simulink model "ACDCMG_woPV"  (R2020b)
settings: Solver=FixedStepAuto  StartTime=0.0  StopTime=0.2  FixedStep=Ts  MaxStep=1e-2  RelTol=1e-3
InitFcn:
  | Set_parameters_R2018
undefined symbols (not defined in the file): D1, D_invs, Delta, dis11, dis14, dis2, dis3, dis4, dis5, dis6, dis8, DiscIntNeverNeededParam, ee_sli_rtmsupport, fn, Fnom, gcbh, H_invs, Ion, Lithium, max_min, P_Load_3, P_nom_inv, Pnom_T1, Pnom_T2, Pnom_T3, Ql_Load_3, R_Load_9, R_Load_DC, Rl, Rls, S, sigbuilder_block, Ts, Ts_Control, Ts_Power, V1_LL_T3, VnInv, Vnom_DC, Vnom_Diesel, Vnom_prim, Vnom_sec, Vnom_ter_AC_DC, Xl, Xls
libraries: powerlib x238, powerlib_meascontrol x103, powerlib_extras x55, simulink x21, pid_lib x4, eeGeneralControl x2, re_lib x1, electricdrivelib x1, eeSinusoidalMeasurementV2 x1, eePowerMeasurement x1
(part 1 of 9)
settings Model: Creator=Leony  LastModifiedBy=Fangyuan
settings SolverCC: ZeroCrossAlgorithm=Adaptive  SolverResetMethod=Robust
settings DataIOCC: LimitDataPoints=on  SaveFormat=Array  ReturnWorkspaceOutputs=off
settings OptimizationCC: LifeSpan=inf
settings DebuggingCC: AlgebraicLoopMsg=none  UnderspecifiedInitializationDetection=Classic  MergeDetectMultiDrivingBlocksExec=none  IgnoredZcDiagnostic=none  SolverPrmCheckMsg=warning  AllowSymbolicDim=off  SFUnexpectedBacktrackingDiag=warning  SFNoUnconditionalDefaultTransitionDiag=warning  SFExecutionAtInitializationDiag=none  ArithmeticOperatorsInVariantConditions=warning
settings HardwareCC: ProdBitPerPointer=32  ProdBitPerSizeT=32  ProdBitPerPtrDiffT=32  ProdLargestAtomicFloat=None  ProdIntDivRoundTo=Undefined  ProdEndianess=Unspecified  ProdWordSize=32  ProdHWDeviceType=32-bit Generic
settings ModelReferenceCC: PropagateSignalLabelsOutOfModel=off
settings SFSimCC: SimUseLocalCustomCode=off  CustomCodeUndefinedFunction=UseInterfaceOnly
settings RTWCC: RTWUseLocalCustomCode=off
settings CodeAppCC: StateflowObjectComments=on
settings GRTTargetCC: TargetLangStandard=C89/C90 (ANSI)
settings ConfigComp: CovMetricSettings=dw  CovSaveCumulativeToWorkspaceVar=on  CovSaveSingleToWorkspaceVar=on  CovExternalEMLEnable=off
settings SimscapeCC: SimscapeNormalizeSystem=off

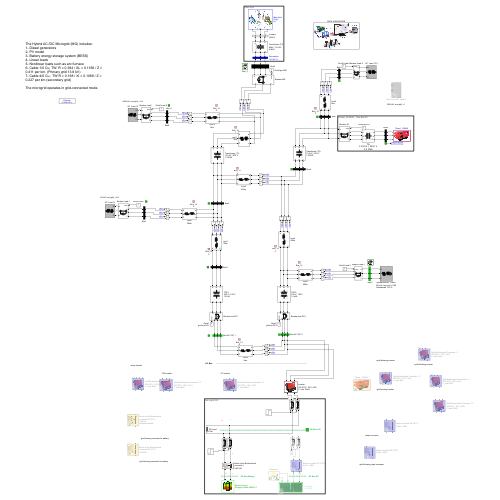
[thumbnail: Simulink's stored preview of the top-level diagram]
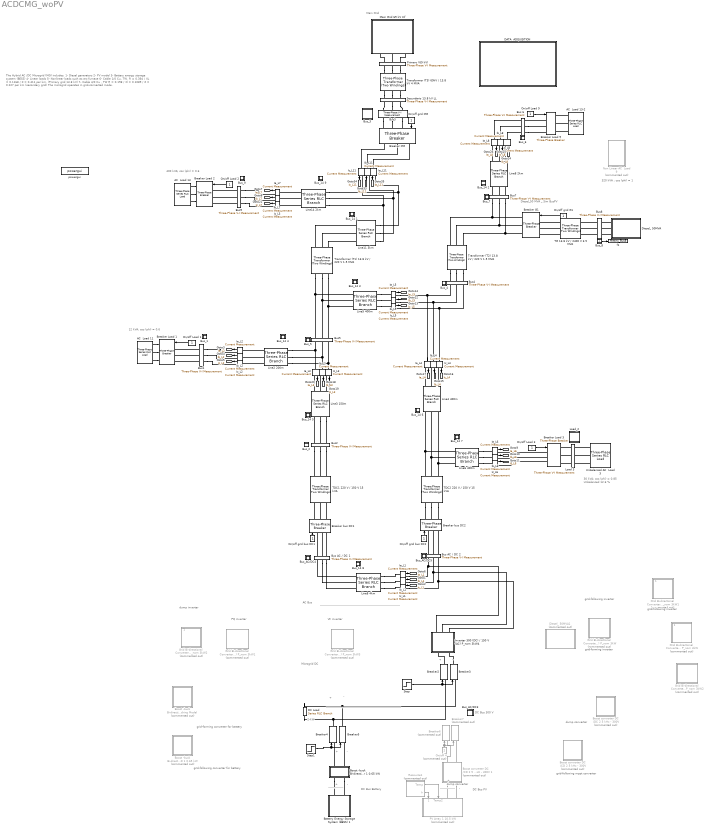
== system ACDCMG_woPV ==
  note: dump inverter
  note: PQ inverter
  note: VF inverter
  note: grid-following inverter
  note: grid-following converter for battery
  note: grid-forming inverter
  note: dump converter
  note: grid-following mppt converter
  note: Main Grid
  note: The Hybrid AC /DC Microgrid (MG) includes:
      | 1- Diesel generators
      | 2- PV model
      | 3- Battery energy storage system (BESS)
      | 4- Linear loads
      | 5- Nonlinear loads such as arc furnace
      | 6- Cable 1/0 Cu, TW. R = 0.394 / XL = 0.1168 / Z = 0.411 per km. (Primary grid 13.8 kV)
      | 7- Cable 4/0 Cu , TW R = 0.198 / Xl = 0.1089 / Z = 0.227 per km (secondary grid)
      |
      | The microgrid operates in grid-connected mode.
  note: --------------------------------------------------------------------------------
  note: AC Bus
  note: Diesel_50 MVA _ Sim BusPV
  note: 30 kVA; cos (phi) = 0.85
      | Unbalanced 12.6 %
  note: 320 kVA ; cos (phi) = 1
  note: 12 kVA; cos (phi) = 0.6
  note: 400 kVA; cos (phi) = 0.6
  note: grid-forming converter for battery
  note: -
  note: ---------------------------------------------------------------------------
  note: -
  note: DC Bus Battery
  note: DC Bus 300 V
  note: +
  note: ---------------
  note: -
  note: -
  note: +
  note: +
  note: 2 kW
  note: +
  note: ---------------
  note: dump converter
  note: DC Bus PV
  note: +
  note: -
  note: Microgrid DC
  note: grid-following inverter
    Ic_L{3..4,8,11} (4 alike) : powerlib/Measurements/Current Measurement  PhasorSimulation=off  OutputType=Complex  PSBequivalent=0
  "  PV Array 1 10.5 kW" : Subsystem  Commented=on
      mask Display: image(imread('Icons\PV.png'));
  " Bus3" : powerlib/Measurements/Three-Phase V-I Measurement  VoltageMeasurement=phase-to-ground  SetLabelV=on  LabelV=Vabc_LL_Bus3  Vpu=off  VpuLL=off  CurrentMeasurement=yes  SetLabelI=on  LabelI=Iabc_LL_Bus3  Ipu=off  Pbase=100e6  Vbase=500e3  OutputType=Complex  PhasorSimulation=off  PSBequivalent=0
  AC  Load 11 : powerlib/Elements/Three-Phase Series RLC Load  LConnTagsString=A|B|C  Configuration=Y (grounded)  NominalVoltage=Vnom_sec  Vabc=[1e3 1e3 1e3]  Vabcp=[1e3 1e3 1e3]  NominalFrequency=Fnom  UnbalancedPower=off  ActivePower=P_Load_11  InductivePower=Ql_Load_11  CapacitivePower=0  Pabc=[10e3 9e3 11e3]  QLabc=[100 90 110]  QCabc=[100 90 110]  Pabcp=[10e3 9e3 11e3]  QLabcp=[100 90 110]  QCabcp=[100 90 110]  Measurements=None  LoadType=constant Z
  AC  Load 13 : powerlib/Elements/Three-Phase Series RLC Load  LConnTagsString=A|B|C  Configuration=Y (grounded)  NominalVoltage=Vnom_prim  Vabc=[1e3 1e3 1e3]  Vabcp=[1e3 1e3 1e3]  NominalFrequency=Fnom  UnbalancedPower=off  ActivePower=P_Load_13  InductivePower=Ql_Load_13  CapacitivePower=0  Pabc=[10e3 9e3 11e3]  QLabc=[100 90 110]  QCabc=[100 90 110]  Pabcp=[10e3 9e3 11e3]  QLabcp=[100 90 110]  QCabcp=[100 90 110]  Measurements=None  LoadType=constant Z
  AC  Load 13-2 : powerlib/Elements/Three-Phase Series RLC Load  LConnTagsString=A|B|C  Configuration=Y (grounded)  NominalVoltage=Vnom_prim  Vabc=[1e3 1e3 1e3]  Vabcp=[1e3 1e3 1e3]  NominalFrequency=Fnom  UnbalancedPower=off  ActivePower=P_Load_15  InductivePower=Ql_Load_15  CapacitivePower=0  Pabc=[10e3 9e3 11e3]  QLabc=[100 90 110]  QCabc=[100 90 110]  Pabcp=[10e3 9e3 11e3]  QLabcp=[100 90 110]  QCabcp=[100 90 110]  Measurements=None  LoadType=constant Z
  Battery Energy Storage System (BESS) 1 : Subsystem
      mask Display: image('Icons\Battery Energy Storage System (BESS).png');
  Boost -buck Bi-directional converter 1 0.65 kW : Subsystem
      mask Display: image(imread('Icons\DC_DC_Converter.jpg'));
  Boost -buck Bi-directional converter DC /CD 1 0.65 kW : Subsystem  Commented=on
      mask Display: image(imread('Icons\DC_DC_Converter.jpg'));
  Boost -buck Bi-directional converter DC /DC 1 0.65 kW Switching Model : Subsystem  Commented=on
      mask Display: image(imread('Icons\DC_DC_Converter.jpg'));
  "Boost converter DC /CD 2 5 kHz - 300V " : Subsystem  Commented=on
      mask Display: image(imread('Icons\DC_DC_Converter.jpg'));
  Boost converter DC /CD 2 5 kHz - 300V 1 : Subsystem  Commented=on
      mask Display: image(imread('Icons\DC_DC_Converter.jpg'));
  "Boost converter DC /DC 2 5 kHz - 300V " : Subsystem  Commented=on
      mask Display: image(imread('Icons\DC_DC_Converter.jpg'));
  Breaker G1 : powerlib/Elements/Three-Phase Breaker  InitialState=closed  SwitchA=on  SwitchB=on  SwitchC=on  SwitchTimes="[4/60  10/60]"  External=on  BreakerResistance=0.001  SnubberResistance=1e6  SnubberCapacitance=inf  Measurements=None
  Breaker Load {1..3,9} (4 alike) : powerlib/Elements/Three-Phase Breaker  InitialState=closed  SwitchA=on  SwitchB=on  SwitchC=on  SwitchTimes="[4/60  10/60]"  External=on  BreakerResistance=0.001  SnubberResistance=1e6  SnubberCapacitance=inf  Measurements=None
  Breaker MG : powerlib/Elements/Three-Phase Breaker  InitialState=closed  SwitchA=on  SwitchB=on  SwitchC=on  SwitchTimes="[4/60  10/60]"  External=on  BreakerResistance=0.001  SnubberResistance=1e6  SnubberCapacitance=inf  Measurements=None
  Breaker bus DC1 : powerlib/Elements/Three-Phase Breaker  InitialState=closed  SwitchA=on  SwitchB=on  SwitchC=on  SwitchTimes="[4/60  10/60]"  External=on  BreakerResistance=0.001  SnubberResistance=1e6  SnubberCapacitance=inf  Measurements=None
  Breaker bus DC2 : powerlib/Elements/Three-Phase Breaker  InitialState=closed  SwitchA=on  SwitchB=on  SwitchC=on  SwitchTimes="[4/60  10/60]"  External=on  BreakerResistance=0.001  SnubberResistance=1e6  SnubberCapacitance=inf  Measurements=None
  Breaker{2..5} (4 alike) : powerlib/Elements/Breaker  InitialState=1  SwitchingTimes="[1/60  5/60]"  External=on  BreakerResistance=0.01  SnubberResistance=1e6  SnubberCapacitance=inf  Measurements=None  MoreParameters=on  NoBreakLoop=off
  Breaker6 : powerlib/Elements/Breaker  Commented=on  InitialState=1  SwitchingTimes="[1/60  5/60]"  External=on  BreakerResistance=0.01  SnubberResistance=1e6  SnubberCapacitance=inf  Measurements=None  MoreParameters=on  NoBreakLoop=off
  Breaker7 : powerlib/Elements/Breaker  Commented=on  InitialState=1  SwitchingTimes="[1/60  5/60]"  External=on  BreakerResistance=0.01  SnubberResistance=1e6  SnubberCapacitance=inf  Measurements=None  MoreParameters=on  NoBreakLoop=off
  Bus 6 : powerlib/Measurements/Three-Phase V-I Measurement  VoltageMeasurement=phase-to-ground  SetLabelV=on  LabelV=VabcLL_Bus_6  Vpu=off  VpuLL=off  CurrentMeasurement=yes  SetLabelI=on  LabelI=IabcLL_Bus_6  Ipu=off  Pbase=100e6  Vbase=25e3/sqrt(2)  OutputType=Complex  PhasorSimulation=off  PSBequivalent=0
  Bus AC / DC 1 : powerlib/Measurements/Three-Phase V-I Measurement  VoltageMeasurement=phase-to-ground  SetLabelV=on  LabelV=Vabc_B1_busDC1  Vpu=off  VpuLL=off  CurrentMeasurement=yes  SetLabelI=on  LabelI=Iabc_B1_busDC1  Ipu=off  Pbase=100e6  Vbase=25e3  OutputType=Complex  PhasorSimulation=off  PSBequivalent=0
  Bus AC / DC 2 : powerlib/Measurements/Three-Phase V-I Measurement  VoltageMeasurement=phase-to-ground  SetLabelV=on  LabelV=Vabc_B1_busDC2  Vpu=off  VpuLL=off  CurrentMeasurement=yes  SetLabelI=on  LabelI=Iabc_B1_busDC2  Ipu=off  Pbase=100e6  Vbase=25e3  OutputType=Complex  PhasorSimulation=off  PSBequivalent=0
  Bus1 : powerlib/Measurements/Three-Phase V-I Measurement  VoltageMeasurement=phase-to-ground  SetLabelV=on  LabelV=VabcLL_Bus_1  Vpu=off  VpuLL=off  CurrentMeasurement=yes  SetLabelI=on  LabelI=IabcLL_Bus_1  Ipu=off  Pbase=100e6  Vbase=380/sqrt(2)  OutputType=Complex  PhasorSimulation=off  PSBequivalent=0
  Bus2 : powerlib/Measurements/Three-Phase V-I Measurement  VoltageMeasurement=phase-to-ground  SetLabelV=on  LabelV=VabcLL_Bus_2  Vpu=off  VpuLL=off  CurrentMeasurement=yes  SetLabelI=on  LabelI=IabcLL_Bus_2  Ipu=off  Pbase=100e6  Vbase=380/sqrt(2)  OutputType=Complex  PhasorSimulation=off  PSBequivalent=0
  Bus4 : powerlib/Measurements/Three-Phase V-I Measurement  VoltageMeasurement=phase-to-ground  SetLabelV=on  LabelV=VabcLL_Bus_4  Vpu=off  VpuLL=off  CurrentMeasurement=yes  SetLabelI=on  LabelI=IabcLL_Bus_4  Ipu=off  Pbase=100e6  Vbase=380/sqrt(2)  OutputType=Complex  PhasorSimulation=off  PSBequivalent=0
  Bus5 : powerlib/Measurements/Three-Phase V-I Measurement  VoltageMeasurement=phase-to-ground  SetLabelV=on  LabelV=VabcLL_Bus_5  Vpu=off  VpuLL=off  CurrentMeasurement=yes  SetLabelI=on  LabelI=IabcLL_Bus_5  Ipu=off  Pbase=100e6  Vbase=380/sqrt(2)  OutputType=Complex  PhasorSimulation=off  PSBequivalent=0
  Bus7 : powerlib/Measurements/Three-Phase V-I Measurement  VoltageMeasurement=phase-to-ground  SetLabelV=on  LabelV=VabcLL_Bus_7  Vpu=off  VpuLL=off  CurrentMeasurement=yes  SetLabelI=on  LabelI=IabcLL_Bus_7  Ipu=off  Pbase=100e6  Vbase=25e3/sqrt(2)  OutputType=Complex  PhasorSimulation=off  PSBequivalent=0
  Bus8 : powerlib/Measurements/Three-Phase V-I Measurement  VoltageMeasurement=phase-to-ground  SetLabelV=on  LabelV=VabcLL_Bus_8  Vpu=off  VpuLL=off  CurrentMeasurement=yes  SetLabelI=on  LabelI=IabcLL_Bus_8  Ipu=off  Pbase=100e6  Vbase=25e3/sqrt(2)  OutputType=Complex  PhasorSimulation=off  PSBequivalent=0
  Bus9 : powerlib/Measurements/Three-Phase V-I Measurement  VoltageMeasurement=phase-to-ground  SetLabelV=on  LabelV=VabcLL_Bus_9  Vpu=off  VpuLL=off  CurrentMeasurement=yes  SetLabelI=on  LabelI=IabcLL_Bus_9  Ipu=off  Pbase=100e6  Vbase=380/sqrt(2)  OutputType=Complex  PhasorSimulation=off  PSBequivalent=0
  Bus_1 : Subsystem
  Bus_14 1 : Subsystem
  Bus_14 2 : Subsystem
  Bus_14 3 : Subsystem
  Bus_14 4 : Subsystem
  Bus_14 5 : Subsystem
  Bus_14 6 : Subsystem
  Bus_14 7 : Subsystem
  Bus_14 8 : Subsystem
  Bus_14 9 : Subsystem
  Bus_2 : Subsystem
  "Bus_3 " : Subsystem
      mask Display: image('Icons\S_meeter.png');
  Bus_4 : Subsystem
  Bus_5 : Subsystem
  Bus_6 : Subsystem
  Bus_7 : Subsystem
  "Bus_8      " : Subsystem
  Bus_9 : Subsystem
  Bus_AC/DC3 : Subsystem
  Bus_AC/DC4 : Subsystem
  Bus_AC/DC5 : Subsystem
  DATA  ADQUISITION : Subsystem
      mask Display: image('Icons\SCADA.png');
  DC Load : powerlib/Elements/Series RLC Branch  LConnTagsString=__new0  RConnTagsString=__new0  BranchType=R  Resistance=R_Load_DC  Inductance=1e-3  SetiL0=off  InitialCurrent=0  Capacitance=1e-6  Setx0=off  InitialVoltage=0  Measurements=None
  Diesel_ 50MVA : Subsystem
      mask Display: image(imread('Icons\Diesel 50kW1.png'));
  Diesel_ 50MVA1 : Subsystem  Commented=on
      mask Display: image(imread('Icons\Diesel 50kW1.png'));
  Grid Bi-directional Converter 1.1 300 (DC) / 150 V (AC) P_nom 3kW : Subsystem  Commented=on
      mask Display: image(imread('Icons\Inverter.png'));
  Grid Bi-directional Converter 1.1 300 (DC) / 150 V (AC) P_nom 3kW1 : Subsystem  Commented=on
      mask Display: image(imread('Icons\Inverter.png'));
  Grid Bi-directional Converter 1.1 300 (DC) / 150 V (AC) P_nom 3kW2 : Subsystem  Commented=on
      mask Display: image(imread('Icons\Inverter.png'));
  Grid Bi-directional Converter 1.2 300 (DC) / 150 V (AC) P_nom 3kW : Subsystem  Commented=on
      mask Display: image(imread('Icons\Inverter.png'));
  Grid Bi-directional Converter 1.2 300 (DC) / 150 V (AC) P_nom 3kW1 : Subsystem  Commented=on
      mask Display: image(imread('Icons\Inverter.png'));
  Grid Bi-directional Converter 1.2 300 (DC) / 150 V (AC) P_nom 3kW2 : Subsystem  Commented=on
      mask Display: image(imread('Icons\Inverter.png'));
  Grid Bi-directional Converter 1.2 300 (DC) / 150 V (AC) P_nom 3kW3 : Subsystem  Commented=on
      mask Display: image(imread('Icons\Inverter.png'));
  Ia_L{1..8,11} (9 alike) : powerlib/Measurements/Current Measurement  PhasorSimulation=off  OutputType=Complex  PSBequivalent=0
  Ib_L{1..8,11} (9 alike) : powerlib/Measurements/Current Measurement  PhasorSimulation=off  OutputType=Complex  PSBequivalent=0
  Ic_L{1..3,5..6} (5 alike) : powerlib/Measurements/Current Measurement  PhasorSimulation=off  OutputType=Complex  PSBequivalent=0
  Inverter 300 (DC) / 150 V (AC) P_nom 3kW4 : Subsystem
      mask Display: image(imread('Icons\Inverter.png'));
  Line11 3km : powerlib/Elements/Three-Phase Series RLC Branch  LConnTagsString=A|B|C  RConnTagsString=A|B|C  BranchType=RL  Resistance=Rl* dis11  Inductance=Xl/377 * dis11  Capacitance=1e-6  Measurements=None
  Line14 2km : powerlib/Elements/Three-Phase Series RLC Branch  LConnTagsString=A|B|C  RConnTagsString=A|B|C  BranchType=RL  Resistance=Rl * dis14  Inductance=Xl/377 * dis14  Capacitance=1e-6  Measurements=None
  Line2 200m : powerlib/Elements/Three-Phase Series RLC Branch  LConnTagsString=A|B|C  RConnTagsString=A|B|C  BranchType=RL  Resistance=Rls * dis2  Inductance=Xls/377 * dis2  Capacitance=1e-6  Measurements=None
  Line3 150m : powerlib/Elements/Three-Phase Series RLC Branch  LConnTagsString=A|B|C  RConnTagsString=A|B|C  BranchType=RL  Resistance=Rls * dis3  Inductance=Xls/377 * dis3  Capacitance=1e-6  Measurements=None
  Line4 400m : powerlib/Elements/Three-Phase Series RLC Branch  LConnTagsString=A|B|C  RConnTagsString=A|B|C  BranchType=RL  Resistance=Rls * dis4  Inductance=Xls/377 * dis4  Capacitance=1e-6  Measurements=None
  Line5 400m : powerlib/Elements/Three-Phase Series RLC Branch  LConnTagsString=A|B|C  RConnTagsString=A|B|C  BranchType=RL  Resistance=Rls * dis5  Inductance=Xls/377 * dis5  Capacitance=1e-6  Measurements=None
  Line6 400m : powerlib/Elements/Three-Phase Series RLC Branch  LConnTagsString=A|B|C  RConnTagsString=A|B|C  BranchType=RL  Resistance=Rls * dis6  Inductance=Xls/377 * dis6  Capacitance=1e-6  Measurements=None
  Line8 2km : powerlib/Elements/Three-Phase Series RLC Branch  LConnTagsString=A|B|C  RConnTagsString=A|B|C  BranchType=RL  Resistance=Rl * dis8  Inductance=Xl/377 * dis8  Capacitance=1e-6  Measurements=None
  Line8 4km : powerlib/Elements/Three-Phase Series RLC Branch  LConnTagsString=A|B|C  RConnTagsString=A|B|C  BranchType=RL  Resistance=Rl * dis5  Inductance=Xl/377 * dis5  Capacitance=1e-6  Measurements=None
  Load 3 : powerlib/Measurements/Three-Phase V-I Measurement  VoltageMeasurement=phase-to-ground  SetLabelV=on  LabelV=Vabc_load_2  Vpu=off  VpuLL=off  CurrentMeasurement=yes  SetLabelI=on  LabelI=Iabc_load_2  Ipu=off  Pbase=100e6  Vbase=380/sqrt(2)  OutputType=Complex  PhasorSimulation=off  PSBequivalent=0
  Load_2 : Subsystem
      mask Display: image('Icons\S_meeter.png');
  Main Grid 69 kV Inf : Subsystem
      mask Display: image('Icons\Main-grid.png');
  Non Linear AC  Load 9 : Subsystem  Commented=on
  On/off grid bus DC1 : Constant
  On/off grid bus DC2 : Constant
  On/off 4 : Constant  Commented=on
  On/off Load {1..3,9} (4 alike) : Constant
  On/off grid G1 : Constant
  On/off grid MG : Constant
  Primary (69 kV) : powerlib/Measurements/Three-Phase V-I Measurement  VoltageMeasurement=phase-to-ground  SetLabelV=on  LabelV=Vabc_Prim_pu  Vpu=off  VpuLL=on  CurrentMeasurement=yes  SetLabelI=on  LabelI=Iabc_Prim  Ipu=on  Pbase=100e6  Vbase=69e3/sqrt(2)  OutputType=Magnitude  PhasorSimulation=off  PSBequivalent=0
  Resource1 : Subsystem  Commented=on
      mask Display: image(imread('Icons\R_Sol.jpg'));
  Secundario 13.8 kV LL : powerlib/Measurements/Three-Phase V-I Measurement  VoltageMeasurement=phase-to-phase  SetLabelV=on  LabelV=Vabc_Sec_pu  Vpu=off  VpuLL=on  CurrentMeasurement=yes  SetLabelI=on  LabelI=Iabc_Sec_pu  Ipu=off  Pbase=250e6  Vbase=Vnom_prim/sqrt(2)  OutputType=Magnitude  PhasorSimulation=off  PSBequivalent=0
  Step : Step  Time=0.1  SampleTime=0  ZeroCross=off
  Step1 : Step  Time=0.001  SampleTime=0  ZeroCross=off
  TDC1 220 V / 150 V 15 kVA : powerlib/Elements/Three-Phase Transformer (Two Windings)  Winding1Connection=Y  Winding2Connection=Y  CoreType=Three single-phase transformers  SetSaturation=off  Hysteresis=off  DataFile='hysteresis'  SetInitialFlux=off  Measurements=None  UNITS=pu  NominalPower=[15e3 , Fnom ]  Winding1=[Vnom_sec , 0.03/2 , 0.03/377]  Winding2=[Vnom_ter_AC_DC , 0.03/2 , 0.03/377]  Rm=500  Lm=500  L0=0.5  Saturation=[ 0,0 ; 0.0024,1.2 ; 1.0,1.52 ]  InitialFluxes=[ 0.8 , -0.8 , 0.7 ]  BreakLoop=off  DiscreteSolver=Trapezoidal iterative  DataType=off  TransfoNumber=1
  TDC2 220 V / 150 V 15 kVA : powerlib/Elements/Three-Phase Transformer (Two Windings)  Winding1Connection=Y  Winding2Connection=Y  CoreType=Three single-phase transformers  SetSaturation=off  Hysteresis=off  DataFile='hysteresis'  SetInitialFlux=off  Measurements=None  UNITS=pu  NominalPower=[15e3 , Fnom ]  Winding1=[Vnom_sec , 0.03/2 , 0.03/377 ]  Winding2=[Vnom_ter_AC_DC , 0.03/2 , 0.03/377 ]  Rm=500  Lm=500  L0=0.5  Saturation=[ 0,0 ; 0.0024,1.2 ; 1.0,1.52 ]  InitialFluxes=[ 0.8 , -0.8 , 0.7 ]  BreakLoop=off  DiscreteSolver=Trapezoidal iterative  DataType=off  TransfoNumber=1
  TG 13.8 kV / 2400 V 3.5 MVA : powerlib/Elements/Three-Phase Transformer (Two Windings)  Winding1Connection=Yg  Winding2Connection=Delta (D1)  CoreType=Three single-phase transformers  SetSaturation=off  Hysteresis=off  DataFile='hysteresis'  SetInitialFlux=off  Measurements=None  UNITS=pu  NominalPower=[3.5e6 , Fnom ]  Winding1=[ Vnom_prim , 0.015/2 , 0.015/2/377]  Winding2=[ Vnom_Diesel , 0.015/2 , 0.015/2/377]  Rm=500  Lm=500  L0=0.5  Saturation="[ 0,0  ;  0.005,1.2  ;  1.0,1.4 ]"  InitialFluxes=[ 0.8 , -0.8 , 0.7 ]  BreakLoop=off  DiscreteSolver=Trapezoidal iterative  DataType=off  TransfoNumber=0
  Transformer (T1) 13.8 kV / 220 V 1.5 MVA : powerlib/Elements/Three-Phase Transformer (Two Windings)  Winding1Connection=Y  Winding2Connection=Y  CoreType=Three single-phase transformers  SetSaturation=off  Hysteresis=off  DataFile='hysteresis'  SetInitialFlux=off  Measurements=None  UNITS=pu  NominalPower=[ Pnom_T1, Fnom ]  Winding1=[Vnom_prim , 0.03/2 , 0.03/(2*377) ]  Winding2=[Vnom_sec , 0.03/2 , 0.03/(2*377) ]  Rm=500  Lm=500  L0=0.5  Saturation=[ 0,0 ; 0.0024,1.2 ; 1.0,1.52 ]  InitialFluxes=[ 0.8 , -0.8 , 0.7 ]  BreakLoop=off  DiscreteSolver=Trapezoidal iterative  DataType=off  TransfoNumber=1
  Transformer (T2) 13.8 kV / 220 V 1.5 MVA : powerlib/Elements/Three-Phase Transformer (Two Windings)  Winding1Connection=Y  Winding2Connection=Y  CoreType=Three single-phase transformers  SetSaturation=off  Hysteresis=off  DataFile='hysteresis'  SetInitialFlux=off  Measurements=None  UNITS=pu  NominalPower=[Pnom_T2 , Fnom]  Winding1=[ Vnom_prim, 0.03/2 , 0.03/(2*377) ]  Winding2=[Vnom_sec , 0.03/2 , 0.03/(2*377) ]  Rm=500  Lm=500  L0=0.5  Saturation=[ 0,0 ; 0.0024,1.2 ; 1.0,1.52 ]  InitialFluxes=[ 0.8 , -0.8 , 0.7 ]  BreakLoop=off  DiscreteSolver=Trapezoidal iterative  DataType=off  TransfoNumber=1
  Transformer (T3) 69kV / 13.8 kV 4 MVA : powerlib/Elements/Three-Phase Transformer (Two Windings)  Winding1Connection=Yg  Winding2Connection=Delta (D1)  CoreType=Three single-phase transformers  SetSaturation=off  Hysteresis=off  DataFile='hysteresis'  SetInitialFlux=off  Measurements=None  UNITS=pu  NominalPower=[Pnom_T3 , Fnom ]  Winding1=[V1_LL_T3 , 0.015/2 , 0.015/(2*377)]  Winding2=[ Vnom_prim, 0.015/2 , 0.015/(2*377)]  Rm=500  Lm=500  L0=0.5  Saturation="[ 0,0  ;  0.005,1.2  ;  1.0,1.4 ]"  InitialFluxes=[ 0.8 , -0.8 , 0.7 ]  BreakLoop=off  DiscreteSolver=Trapezoidal iterative  DataType=off  TransfoNumber=0
  Unbalanced AC  Load 3 : powerlib/Elements/Three-Phase Series RLC Load  LConnTagsString=A|B|C  Configuration=Y (grounded)  NominalVoltage=Vnom_sec  Vabc=[Vnom_sec/sqrt(3), Vnom_sec/sqrt(3), Vnom_sec/sqrt(3)]  Vabcp=[1e3 1e3 1e3]  NominalFrequency=Fnom  UnbalancedPower=on  ActivePower=P_Load_3  InductivePower=Ql_Load_3  CapacitivePower=0  Pabc=[P_Load_3*1.04, P_Load_3, P_Load_3*0.9]  QLabc=[Ql_Load_3*1.04, Ql_Load_3, Ql_Load_3*0.9]  QCabc=[0 0 0]  Pabcp=[10e3 9e3 11e3]  QLabcp=[100 90 110]  QCabcp=[100 90 110]  Measurements=None  LoadType=constant Z
  f1 : ToWorkspace  VariableName=Means_Bus8  SaveFormat=Timeseries  SampleTime=-1
  powergui : powerlib/powergui  Priority=1  SimulationMode=Discrete  SampleTime=Ts_Power  frequency=60  Iterations=50  frequencyindice=0  Pbase=100e6  ErrMax=1e-4  UnitsV=kV  UnitsW=MW  buscounter=0  FunctionMessages=off  echomessages=off  EnableUseOfTLC=off  CurrentSourceSwitches=off  DisableSnubberDevices=off  DisableRonSwitches=off  DisableVfSwitches=off  DisplayEquations=off  AutomaticDiscreteSolvers=off  SolverType=Tustin  Interpol=off  ExternalGateDelay=off  methode=off  Ts=0  x0status=blocks  SPID=off  SwTol=0  HookPort=off  NonlinearTolerance=1e-4  nMaxIteration=100  ContinueOnMaxIteration=off  RestoreLinks=warning  ResistiveCurrentMeasurement=off  Frange=[0:2:500]  Ylog=off  Xlog=on  ShowGrid=off  save=off  variable=ZData  structure=0  ZoomFFT=off  StartTime=0.0  cycles=1  DisplayStyle=1  fundamental=60  FreqAxis=off  MaxFrequency=1000  frequencyindicesteady=1  RmsSteady=1  display=off
  tag scope: Ia_L11=global, Ia_L1=global, Ia_L2=global, Ia_L3=global, Ia_L4=global, Ia_L5=global, Ia_L6=global, Ia_L7=global, Ia_L8=global, Ib_L11=global, Ib_L1=global, Ib_L2=global, Ib_L3=global, Ib_L4=global, Ib_L5=global, Ib_L6=global, Ib_L7=global, Ib_L8=global, Ic_L11=global, Ic_L1=global, Ic_L2=global, Ic_L3=global, Ic_L4=global, Ic_L5=global, Ic_L6=global, Ic_L7=global, Ic_L8=global
  wires:
  On/off grid MG/1 -> Breaker MG/1
  On/off Load 9/1 -> Breaker Load 9/1
  Ib_L2/1 -> [Ib_L2]
  Ia_L2/1 -> [Ia_L2]
  Ic_L2/1 -> [Ic_L2]
  Ic_L6/1 -> [Ic_L6]
  Ia_L6/1 -> [Ia_L6]
  Ib_L6/1 -> [Ib_L6]
  Ic_L5/1 -> [Ic_L5]
  Ib_L5/1 -> [Ib_L5]
  Ia_L5/1 -> [Ia_L5]
  Ia_L4/1 -> [Ia_L4]
  Ib_L4/1 -> [Ib_L4]
  "  Ic_L4"/1 -> [Ic_L4]
  "  Ic_L3"/1 -> [Ic_L3]
  Ib_L3/1 -> [Ib_L3]
  Ia_L3/1 -> [Ia_L3]
  Ia_L8/1 -> [Ia_L8]
  Ib_L8/1 -> [Ib_L8]
  "  Ic_L8"/1 -> [Ic_L8]
  "  Ic_L11"/1 -> [Ic_L11]
  Ib_L11/1 -> [Ib_L11]
  Ia_L11/1 -> [Ia_L11]
  On/off grid bus DC1/1 -> Breaker bus DC1/1
  On/off grid bus DC2/1 -> Breaker bus DC2/1
  "Bus_8      "/1("Means_Bus8      ") -> f1/1
  On/off grid G1/1 -> Breaker G1/1
  On/off Load 3/1 -> Breaker Load 3/1
  On/off Load 1/1 -> Breaker Load 1/1
  Ic_L1/1 -> [Ic_L1]
  Ib_L1/1 -> [Ib_L1]
  Ia_L1/1 -> [Ia_L1]
  On/off Load 2/1 -> Breaker Load 2/1
  Ib_L7/1 -> [Ib_L7]
  Ic_L3/1 -> [Ic_L7]
  Ia_L7/1 -> [Ia_L7]
  Resource1/2(Ir) -> "  PV Array 1 10.5 kW"/1(Irradiance)
  Step1/1 -> Breaker5/1, Breaker4/1
  Step/1 -> Breaker3/1, Breaker2/1
  Resource1/1(Temp) -> "  PV Array 1 10.5 kW"/2(Temp2)
  On/off 4/1 -> Breaker7/1, Breaker6/1
  connections:
  Bus1/RConn3 -- Ic_L2/RConn1
  Bus1/RConn2 -- Ib_L2/RConn1
  Bus1/RConn1 -- Ia_L2/RConn1
  Bus2/LConn1 -- TDC1 220 V / 150 V 15 kVA/LConn1
  Bus2/LConn2 -- TDC1 220 V / 150 V 15 kVA/LConn2
  Bus2/LConn3 -- TDC1 220 V / 150 V 15 kVA/LConn3
  Ia_L3/LConn1 -- Line2 200m/RConn1 -- Bus5/RConn1
  Ib_L3/LConn1 -- Line2 200m/RConn2 -- Bus5/RConn2
  "  Ic_L3"/LConn1 -- Line2 200m/RConn3 -- Bus5/RConn3
  Line4 400m/LConn2 -- Line6 400m/LConn2 -- TDC2 220 V / 150 V 15 kVA/LConn2
  TDC2 220 V / 150 V 15 kVA/LConn3 -- Line6 400m/LConn3 -- Line4 400m/LConn3
  Ia_L4/LConn1 -- Ia_L5/RConn1 -- Bus4/RConn1
  Ib_L4/LConn1 -- Ib_L5/RConn1 -- Bus4/RConn2
  "  Ic_L4"/LConn1 -- Ic_L5/RConn1 -- Bus4/RConn3
  Transformer (T1) 13.8 kV / 220 V 1.5 MVA/RConn1 -- Line5 400m/LConn1 -- Bus5/LConn1
  Transformer (T1) 13.8 kV / 220 V 1.5 MVA/RConn2 -- Line5 400m/LConn2 -- Bus5/LConn2
  Transformer (T1) 13.8 kV / 220 V 1.5 MVA/RConn3 -- Line5 400m/LConn3 -- Bus5/LConn3
  Breaker Load 3/LConn1 -- Ia_L6/RConn1
  Breaker Load 3/LConn2 -- Ib_L6/RConn1
  Breaker Load 3/LConn3 -- Ic_L6/RConn1
  Line11 3km/LConn1 -- Transformer (T1) 13.8 kV / 220 V 1.5 MVA/LConn1
  Line11 3km/LConn2 -- Transformer (T1) 13.8 kV / 220 V 1.5 MVA/LConn2
  Line11 3km/LConn3 -- Transformer (T1) 13.8 kV / 220 V 1.5 MVA/LConn3
  Ia_L11/LConn1 -- Breaker MG/RConn1
  Ib_L11/LConn1 -- Breaker MG/RConn2
  "  Ic_L11"/LConn1 -- Breaker MG/RConn3
  Transformer (T2) 13.8 kV / 220 V 1.5 MVA/RConn1 -- Bus4/LConn1
  Transformer (T2) 13.8 kV / 220 V 1.5 MVA/RConn2 -- Bus4/LConn2
  Transformer (T2) 13.8 kV / 220 V 1.5 MVA/RConn3 -- Bus4/LConn3
  Breaker G1/RConn1 -- Bus7/LConn1 -- Transformer (T2) 13.8 kV / 220 V 1.5 MVA/LConn1
  Breaker G1/RConn2 -- Bus7/LConn2 -- Transformer (T2) 13.8 kV / 220 V 1.5 MVA/LConn2
  Breaker G1/RConn3 -- Bus7/LConn3 -- Transformer (T2) 13.8 kV / 220 V 1.5 MVA/LConn3
  Primary (69 kV)/LConn2 -- Main Grid 69 kV Inf/RConn2
  Transformer (T3) 69kV / 13.8 kV 4 MVA/RConn1 -- Secundario 13.8 kV LL/LConn1
  Primary (69 kV)/RConn3 -- Transformer (T3) 69kV / 13.8 kV 4 MVA/LConn3
  Primary (69 kV)/RConn1 -- Transformer (T3) 69kV / 13.8 kV 4 MVA/LConn1
  Transformer (T3) 69kV / 13.8 kV 4 MVA/RConn2 -- Secundario 13.8 kV LL/LConn2
  Primary (69 kV)/LConn1 -- Main Grid 69 kV Inf/RConn3
  Transformer (T3) 69kV / 13.8 kV 4 MVA/RConn3 -- Secundario 13.8 kV LL/LConn3
  Primary (69 kV)/LConn3 -- Main Grid 69 kV Inf/RConn1
  Primary (69 kV)/RConn2 -- Transformer (T3) 69kV / 13.8 kV 4 MVA/LConn2
  Line4 400m/LConn1 -- Line6 400m/LConn1 -- TDC2 220 V / 150 V 15 kVA/LConn1
  Secundario 13.8 kV LL/RConn3 -- " Bus3"/LConn3
  Secundario 13.8 kV LL/RConn2 -- " Bus3"/LConn2
  Secundario 13.8 kV LL/RConn1 -- " Bus3"/LConn1
  " Bus3"/RConn3 -- Breaker MG/LConn3
  " Bus3"/RConn2 -- Breaker MG/LConn2
  " Bus3"/RConn1 -- Breaker MG/LConn1
  Line2 200m/LConn1 -- Ia_L2/LConn1
  Line2 200m/LConn2 -- Ib_L2/LConn1
  Line2 200m/LConn3 -- Ic_L2/LConn1
  Line6 400m/RConn1 -- Ia_L6/LConn1
  Line6 400m/RConn2 -- Ib_L6/LConn1
  Line6 400m/RConn3 -- Ic_L6/LConn1
  Line5 400m/RConn1 -- Ia_L5/LConn1
  Line5 400m/RConn2 -- Ib_L5/LConn1
  Line5 400m/RConn3 -- Ic_L5/LConn1
  Line4 400m/RConn1 -- Ia_L4/RConn1
  Line4 400m/RConn2 -- Ib_L4/RConn1
  Line4 400m/RConn3 -- "  Ic_L4"/RConn1
  Line3 150m/RConn1 -- Ia_L3/RConn1
  Line3 150m/RConn2 -- Ib_L3/RConn1
  Line3 150m/RConn3 -- "  Ic_L3"/RConn1
  Line8 2km/RConn1 -- Ia_L8/RConn1
  Line8 2km/RConn2 -- Ib_L8/RConn1
  Line8 2km/RConn3 -- "  Ic_L8"/RConn1
  Line11 3km/RConn3 -- Line14 2km/RConn3 -- "  Ic_L11"/RConn1
  Line11 3km/RConn2 -- Line14 2km/RConn2 -- Ib_L11/RConn1
  Line11 3km/RConn1 -- Line14 2km/RConn1 -- Ia_L11/RConn1
  TDC2 220 V / 150 V 15 kVA/RConn3 -- Breaker bus DC2/RConn3
  Breaker bus DC1/RConn2 -- TDC1 220 V / 150 V 15 kVA/RConn2
  TDC2 220 V / 150 V 15 kVA/RConn2 -- Breaker bus DC2/RConn2
  Breaker bus DC1/RConn1 -- TDC1 220 V / 150 V 15 kVA/RConn1
  TDC2 220 V / 150 V 15 kVA/RConn1 -- Breaker bus DC2/RConn1
  Breaker bus DC1/RConn3 -- TDC1 220 V / 150 V 15 kVA/RConn3
  Ic_L1/RConn1 -- Inverter 300 (DC) / 150 V (AC) P_nom 3kW4/LConn3 -- Bus AC / DC 2/LConn3
  Ia_L1/RConn1 -- Inverter 300 (DC) / 150 V (AC) P_nom 3kW4/LConn1 -- Bus AC / DC 2/LConn1
  Bus AC / DC 1/RConn2 -- Breaker bus DC1/LConn2
  Bus AC / DC 2/RConn3 -- Breaker bus DC2/LConn3
  Line8 4km/LConn1 -- Bus AC / DC 1/LConn1
  Bus AC / DC 2/RConn1 -- Breaker bus DC2/LConn1
  Bus AC / DC 1/RConn1 -- Breaker bus DC1/LConn1
  Bus AC / DC 2/RConn2 -- Breaker bus DC2/LConn2
  Bus AC / DC 1/RConn3 -- Breaker bus DC1/LConn3
  TG 13.8 kV / 2400 V 3.5 MVA/LConn1 -- Breaker G1/LConn1
  TG 13.8 kV / 2400 V 3.5 MVA/LConn3 -- Breaker G1/LConn3
  Diesel_ 50MVA/LConn1 -- Bus8/LConn1
  Bus8/RConn1 -- TG 13.8 kV / 2400 V 3.5 MVA/RConn1
  Diesel_ 50MVA/LConn2 -- Bus8/LConn2
  TG 13.8 kV / 2400 V 3.5 MVA/LConn2 -- Breaker G1/LConn2
  Diesel_ 50MVA/LConn3 -- Bus8/LConn3
  Bus8/RConn2 -- TG 13.8 kV / 2400 V 3.5 MVA/RConn2
  Bus8/RConn3 -- TG 13.8 kV / 2400 V 3.5 MVA/RConn3
  Load 3/LConn3 -- Breaker Load 3/RConn3
  Load 3/LConn1 -- Breaker Load 3/RConn1
  Unbalanced AC  Load 3/LConn3 -- Load 3/RConn3
  Unbalanced AC  Load 3/LConn1 -- Load 3/RConn1
  Load 3/LConn2 -- Breaker Load 3/RConn2
  Unbalanced AC  Load 3/LConn2 -- Load 3/RConn2
  Bus 6/LConn1 -- Ia_L8/LConn1
  Bus 6/LConn2 -- Ib_L8/LConn1
  Bus 6/LConn3 -- "  Ic_L8"/LConn1
  Bus 6/RConn3 -- Breaker Load 9/LConn3
  Bus 6/RConn2 -- Breaker Load 9/LConn2
  Breaker Load 9/LConn1 -- Bus 6/RConn1
  Bus7/RConn1 -- Line8 2km/LConn1
  Bus7/RConn2 -- Line8 2km/LConn2
  Bus7/RConn3 -- Line8 2km/LConn3
  Line3 150m/LConn3 -- Bus2/RConn3
  Line3 150m/LConn2 -- Bus2/RConn2
  Bus2/RConn1 -- Line3 150m/LConn1
  AC  Load 11/LConn1 -- Breaker Load 1/RConn1
  Bus1/LConn2 -- Breaker Load 1/LConn2
  AC  Load 11/LConn3 -- Breaker Load 1/RConn3
  AC  Load 11/LConn2 -- Breaker Load 1/RConn2
  Bus1/LConn3 -- Breaker Load 1/LConn3
  Bus1/LConn1 -- Breaker Load 1/LConn1
  Line8 4km/RConn3 -- Ic_L1/LConn1
  Line8 4km/RConn1 -- Ia_L1/LConn1
  Line8 4km/RConn2 -- Ib_L1/LConn1
  Bus AC / DC 1/LConn2 -- Line8 4km/LConn2
  Bus AC / DC 1/LConn3 -- Line8 4km/LConn3
  Line14 2km/LConn2 -- Ib_L7/LConn1
  AC  Load 13/LConn2 -- Breaker Load 2/RConn2
  Bus9/RConn1 -- Ia_L7/RConn1
  Bus9/LConn2 -- Breaker Load 2/LConn2
  Bus9/LConn3 -- Breaker Load 2/LConn3
  Line14 2km/LConn1 -- Ia_L7/LConn1
  AC  Load 13/LConn1 -- Breaker Load 2/RConn1
  Bus9/LConn1 -- Breaker Load 2/LConn1
  Line14 2km/LConn3 -- Ic_L3/LConn1
  Bus9/RConn3 -- Ic_L3/RConn1
  Bus9/RConn2 -- Ib_L7/RConn1
  AC  Load 13/LConn3 -- Breaker Load 2/RConn3
  Breaker3/LConn1 -- DC Load/RConn1 -- Breaker5/RConn1
  DC Load/LConn1 -- Breaker2/LConn1 -- Breaker4/RConn1
  Boost converter DC /CD 2 5 kHz - 300V 1/LConn2 -- Breaker7/LConn1
  Boost -buck Bi-directional converter 1 0.65 kW/LConn2 -- Battery Energy Storage System (BESS) 1/LConn2
  Boost converter DC /CD 2 5 kHz - 300V 1/LConn1 -- Breaker6/LConn1
  Boost -buck Bi-directional converter 1 0.65 kW/RConn2 -- Breaker5/LConn1
  Boost -buck Bi-directional converter 1 0.65 kW/LConn1 -- Battery Energy Storage System (BESS) 1/LConn1
  Boost converter DC /CD 2 5 kHz - 300V 1/RConn1 -- "  PV Array 1 10.5 kW"/LConn1
  Boost -buck Bi-directional converter 1 0.65 kW/RConn1 -- Breaker4/LConn1
  Boost converter DC /CD 2 5 kHz - 300V 1/RConn2 -- "  PV Array 1 10.5 kW"/LConn2
  Breaker3/RConn1 -- Inverter 300 (DC) / 150 V (AC) P_nom 3kW4/RConn2
  AC  Load 13-2/LConn1 -- Breaker Load 9/RConn1
  AC  Load 13-2/LConn2 -- Breaker Load 9/RConn2
  AC  Load 13-2/LConn3 -- Breaker Load 9/RConn3
  Ib_L1/RConn1 -- Inverter 300 (DC) / 150 V (AC) P_nom 3kW4/LConn2 -- Bus AC / DC 2/LConn2
  Breaker2/RConn1 -- Inverter 300 (DC) / 150 V (AC) P_nom 3kW4/RConn1

== system ACDCMG_woPV/  PV Array 1 10.5 kW ==
  note: DC Bus
  note: 10.5 - kW  PV Array
      | 42 * SunTech STP - 250S-20 /Wd  (Nser=6 Npar=7)
  Irradiance : Inport
  Temp2 : Inport  Port=2
  PV Array : re_lib/Solar/PV Array  Npar=7  Nser=6  PlotType=array @ 1000 W/m2 & specified temperatures  S_vec="[ 1000  250 ]"  Temp_C_vec="[0 25 50  ]"  ModuleName=User-defined  PlotWhenSelected=off  Pm=250.205  Ncell=96  Voc=37.4  Isc=8.63  Vm=30.7  Im=8.15  beta_Voc_pc=-0.34  alpha_Isc_pc=0.050  beta_Voc=-0.12716  alpha_Isc=0.004315  IL=8.6686  I0=1.3965e-10  nI=0.6105  Rsh=311.9016  Rs=0.26776  RobustModel=off  RobustCellTemperature=313.3991  BAL=on  Tc=Tc  Tfilter=5e-5
  + : PMIOPort  Tag=PMCPort  Side=Left
  - : PMIOPort  Tag=PMCPort  Port=2  Side=Left
  tag scope: m_PV=global
  wires:
  Temp2/1 -> PV Array/2
  Irradiance/1 -> PV Array/1
  PV Array/1 -> [m_PV]
  connections:
  PV Array/RConn1 -- +/RConn1
  PV Array/RConn2 -- -/RConn1

== system ACDCMG_woPV/Battery Energy Storage System (BESS) 1 ==
  Battery1 : electricdrivelib/Extra Sources/Battery  BatType=Lithium-Ion  ShowTempParam=off  ThermalPreset=no  ShowAgeParam=off  NomV=120  NomQ=800  SOC=80  Batt_Tr=3  PresetModel=on  MaxQ=800  MinV=90  FullV=139.6785  Dis_rate=347.8261  R=0.0015  Normal_OP=723.4783  expZone="[129.6463      39.30435]"  current=[30 35 40 46]  Units=Time  Tci=20  NomT=25  T2=0  MaxQ2=2.208  FullV2=3.45  Normal_OP2=2.8  expZone2="[3.22        0.23]"  Rca=0.6  ti=1000  Dp=0  Neq0=0  Tsim=1e6  Ta1=25  Qeol=5.4*0.9  Reol=0.013333*1.2  Char_age=[2.3478, 3]  Dis_age=[2.3478, 10]  N1=1500  N2=10500  N3=1000  N4=1400  Ta2=45  N5=950
  + B1 : PMIOPort  Side=Left
  - B1 : PMIOPort  Port=2  Side=Left
  connections:
  Battery1/LConn2 -- - B1/RConn1
  Battery1/LConn1 -- + B1/RConn1

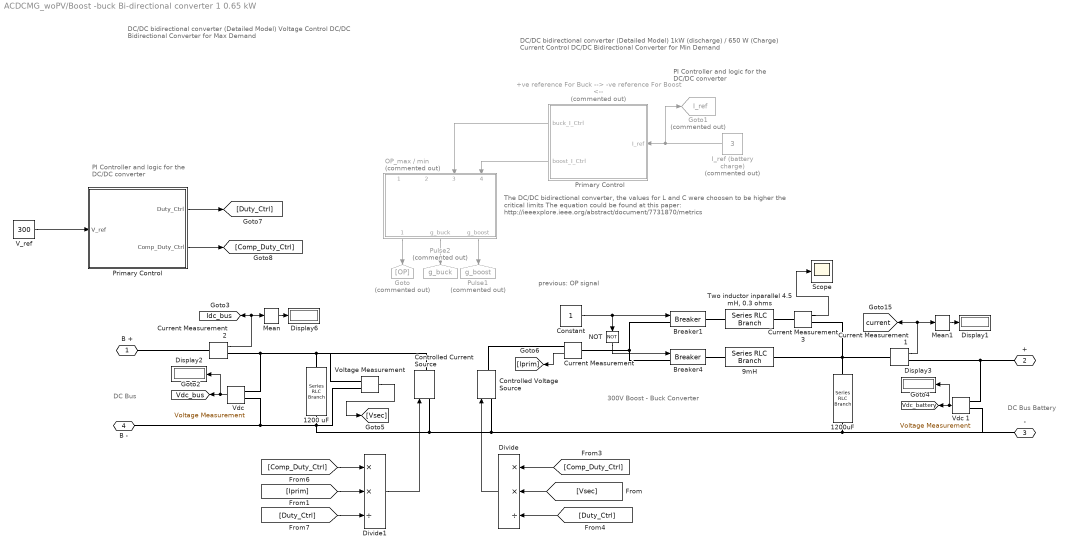
== system ACDCMG_woPV/Boost -buck Bi-directional converter 1 0.65 kW ==
  note: previous: OP signal
  note: Primary Control
  note: DC Bus
  note: DC Bus Battery
  note: PI Controller and logic for
      | the DC/DC converter
  note: DC/DC bidirectional converter (Detailed Model)
      | Voltage Control DC/DC Bidirectional Converter for Max Demand
  note: 300V
      | Boost - Buck Converter
  note: PI Controller and logic for
      | the DC/DC converter
  note: DC/DC bidirectional converter (Detailed Model)
      | 1kW (discharge) / 650 W (Charge)
      | Current Control DC/DC Bidirectional Converter for Min Demand
  note: The DC/DC bidirectional converter, the values for L and C were choosen to be higher the critical limits The equation could be found at this paper:
      | http://ieeexplore.ieee.org/abstract/document/7731870/metrics
  +ve reference For Buck --> -ve reference For Boost <-- : Subsystem  Commented=on
      mask Display: image('Icons\FPGA.png');
  1200 uF : powerlib/Elements/Series RLC Branch  LConnTagsString=__new0  RConnTagsString=__new0  BranchType=RC  Resistance=0.1  Inductance=3e-3  SetiL0=off  InitialCurrent=0  Capacitance=120e-6  Setx0=on  InitialVoltage=300  Measurements=None
  1200uF : powerlib/Elements/Series RLC Branch  LConnTagsString=__new0  RConnTagsString=__new0  BranchType=C  Resistance=1  Inductance=3e-3  SetiL0=off  InitialCurrent=0  Capacitance=1200e-6  Setx0=on  InitialVoltage=120  Measurements=None
  9mH : powerlib/Elements/Series RLC Branch  LConnTagsString=__new0  RConnTagsString=__new0  BranchType=L  Resistance=1  Inductance=9e-3  SetiL0=off  InitialCurrent=0  Capacitance=1e-6  Setx0=off  InitialVoltage=0  Measurements=None
  Breaker1 : powerlib/Elements/Breaker  InitialState=0  SwitchingTimes="[1/60  5/60]"  External=on  BreakerResistance=0.0001  SnubberResistance=1e6  SnubberCapacitance=inf  Measurements=None  MoreParameters=on  NoBreakLoop=off
  Breaker4 : powerlib/Elements/Breaker  InitialState=0  SwitchingTimes="[1/60  5/60]"  External=on  BreakerResistance=0.0001  SnubberResistance=1e6  SnubberCapacitance=inf  Measurements=None  MoreParameters=on  NoBreakLoop=off
  Constant : Constant
  Controlled Current Source : powerlib/Electrical Sources/Controlled Current Source  Initialize=on  Source_Type=AC  Amplitude=0  Phase=0  Frequency=0  Measurements=None
  Controlled Voltage Source : powerlib/Electrical Sources/Controlled Voltage Source  Initialize=on  Source_Type=DC  Amplitude=0  Phase=0  Frequency=0  Measurements=None
  Current Measurement{,1..3} (4 alike) : powerlib/Measurements/Current Measurement  PhasorSimulation=off  OutputType=Complex  PSBequivalent=0
  Display{1..3,6} (4 alike) : Display
  Divide : Product  Inputs=**/
  Divide1 : Product  Inputs=**/
  Goto : Goto  Commented=on  GotoTag=OP
  Goto1 : Goto  Commented=on  GotoTag=I_ref  TagVisibility=global
  I_ref (battery charge) : Constant  Commented=on  Value=3
  Mean : powerlib_meascontrol/Measurements/Mean  Freq=10  Vinit=0  Ts=0
  Mean1 : powerlib_meascontrol/Measurements/Mean  Freq=10  Vinit=0  Ts=0
  NOT : Logic  Operator=NOT  IconShape=distinctive  AllPortsSameDT=off  OutDataTypeStr=boolean
  OP_max / min : Subsystem  Commented=on
  Primary Control : Subsystem
      mask Display: image('Icons\FPGA.png');
  Pulse1 : Goto  Commented=on  GotoTag=g_boost  TagVisibility=global
  Pulse2 : Goto  Commented=on  GotoTag=g_buck  TagVisibility=global
  Scope : Scope
  "Two inductor inparallel 4.5 mH, 0.3 ohms" : powerlib/Elements/Series RLC Branch  LConnTagsString=__new0  RConnTagsString=__new0  BranchType=RL  Resistance=0.3  Inductance=4.5e-5  SetiL0=off  InitialCurrent=0  Capacitance=1e-6  Setx0=off  InitialVoltage=0  Measurements=None
  V_ref : Constant  Value=300
  "Vdc " : powerlib/Measurements/Voltage Measurement  Tag=PoWeRsYsTeMmEaSuReMeNt  PhasorSimulation=off  OutputType=Magnitude  PSBequivalent=0
  Vdc 1 : powerlib/Measurements/Voltage Measurement  Tag=PoWeRsYsTeMmEaSuReMeNt  PhasorSimulation=off  OutputType=Magnitude  PSBequivalent=0
  Voltage Measurement : powerlib/Measurements/Voltage Measurement  PhasorSimulation=off  OutputType=Complex  PSBequivalent=0
  B + : PMIOPort  Side=Right
  + : PMIOPort  Port=2  Side=Left
  - : PMIOPort  Port=3  Side=Left
  B - : PMIOPort  Port=4  Side=Right
  tag scope: Idc_bus=global, Vdc_battery=global, Vdc_bus=global, current=global
  wires:
  "Vdc "/1 -> Display2/1, [Vdc_bus]
  Vdc 1/1 -> Display3/1, [Vdc_battery]
  Current Measurement2/1 -> Mean/1, [Idc_bus]
  Mean/1 -> Display6/1
  Current Measurement1/1 -> [current], Mean1/1
  Mean1/1 -> Display1/1
  V_ref/1 -> Primary Control/1(V_ref)
  OP_max / min/1(Op_Max / Min) -> Goto/1
  Constant/1 -> NOT/1, Breaker1/1
  NOT/1 -> Breaker4/1
  I_ref (battery charge)/1 -> Goto1/1, +ve reference For Buck --> -ve reference For Boost <--/1(I_ref)
  +ve reference For Buck --> -ve reference For Boost <--/1(buck_I_Ctrl) -> OP_max / min/3(buck_I_Ctrl)
  +ve reference For Buck --> -ve reference For Boost <--/2(boost_I_Ctrl) -> OP_max / min/4(boost_I_Ctrll)
  OP_max / min/2(g_buck) -> Pulse2/1
  OP_max / min/3(g_boost) -> Pulse1/1
  Current Measurement3/1 -> Scope/1
  Voltage Measurement/1 -> [Vsec]
  Current Measurement/1 -> [Iprim]
  Primary Control/1(Duty_Ctrl) -> [Duty_Ctrl]
  Primary Control/2(Comp_Duty_Ctrl) -> [Comp_Duty_Ctrl]
  [Vsec] -> Divide/2
  Divide/1 -> Controlled Voltage Source/1
  [Comp_Duty_Ctrl] -> Divide1/1
  [Iprim] -> Divide1/2
  [Duty_Ctrl] -> Divide1/3
  Divide1/1 -> Controlled Current Source/1
  [Comp_Duty_Ctrl] -> Divide/1
  [Duty_Ctrl] -> Divide/3
  connections:
  +/RConn1 -- Vdc 1/LConn1 -- Current Measurement1/RConn1
  Current Measurement/LConn1 -- Breaker4/LConn1 -- Breaker1/LConn1
  "Vdc "/LConn1 -- Current Measurement2/RConn1 -- 1200 uF/LConn1 -- Controlled Current Source/RConn1 -- Voltage Measurement/LConn1
  Voltage Measurement/LConn2 -- "Vdc "/LConn2 -- B -/RConn1 -- 1200 uF/RConn1 -- Controlled Voltage Source/LConn1 -- Vdc 1/LConn2 -- -/RConn1 -- 1200uF/RConn1 -- Controlled Current Source/LConn1
  Current Measurement2/LConn1 -- B +/RConn1
  "Two inductor inparallel 4.5 mH, 0.3 ohms"/LConn1 -- Breaker1/RConn1
  Current Measurement1/LConn1 -- Current Measurement3/RConn1 -- 1200uF/LConn1 -- 9mH/RConn1
  9mH/LConn1 -- Breaker4/RConn1
  "Two inductor inparallel 4.5 mH, 0.3 ohms"/RConn1 -- Current Measurement3/LConn1
  Current Measurement/RConn1 -- Controlled Voltage Source/RConn1

== system ACDCMG_woPV/Boost -buck Bi-directional converter DC //CD 1 0.65 kW ==
  note: DC Bus
  note: DC Bus Battery
  note: PI Controller and logic for
      | the DC/DC converter
  note: DC/DC bidirectional converter (Detailed Model)
      | 1kW (discharge) / 650 W (Charge)
  note: 300V
      | Boost - Buck Converter
  note: The DC/DC bidirectional converter, the values for L and C were choosen to be higher the critical limits The equation could be found at this paper:
      | http://ieeexplore.ieee.org/abstract/document/7731870/metrics
  +ve reference For Buck --> -ve reference For Boost <-- : Subsystem
      mask Display: image('Icons\FPGA.png');
  1200 uF : powerlib/Elements/Series RLC Branch  LConnTagsString=__new0  RConnTagsString=__new0  BranchType=RC  Resistance=0.1  Inductance=3e-3  SetiL0=off  InitialCurrent=0  Capacitance=1200e-6  Setx0=off  InitialVoltage=150  Measurements=None
  1200uF : powerlib/Elements/Series RLC Branch  LConnTagsString=__new0  RConnTagsString=__new0  BranchType=C  Resistance=1  Inductance=3e-3  SetiL0=off  InitialCurrent=0  Capacitance=1200e-6  Setx0=off  InitialVoltage=130  Measurements=None
  1mH1 : powerlib/Elements/Series RLC Branch  LConnTagsString=__new0  RConnTagsString=__new0  BranchType=L  Resistance=1  Inductance=1e-4  SetiL0=off  InitialCurrent=0  Capacitance=1e-6  Setx0=off  InitialVoltage=0  Measurements=None
  9mH : powerlib/Elements/Series RLC Branch  LConnTagsString=__new0  RConnTagsString=__new0  BranchType=L  Resistance=1  Inductance=9e-3  SetiL0=off  InitialCurrent=0  Capacitance=1e-6  Setx0=off  InitialVoltage=0  Measurements=None
  Current Measurement1 : powerlib/Measurements/Current Measurement  PhasorSimulation=off  OutputType=Complex  PSBequivalent=0
  Current Measurement2 : powerlib/Measurements/Current Measurement  PhasorSimulation=off  OutputType=Complex  PSBequivalent=0
  Diode5 : powerlib/Power Electronics/IGBT//Diode  Ron=1e-3  Rs=1e5  Cs=inf  Measurements=on
  Diode6 : powerlib/Power Electronics/IGBT//Diode  Ron=1e-3  Rs=1e5  Cs=inf  Measurements=on
  Display{1..3,6} (4 alike) : Display
  Mean : powerlib_meascontrol/Measurements/Mean  Freq=100  Vinit=0  Ts=0
  Mean1 : powerlib_meascontrol/Measurements/Mean  Freq=10  Vinit=0  Ts=0
  "Vdc " : powerlib/Measurements/Voltage Measurement  Tag=PoWeRsYsTeMmEaSuReMeNt  PhasorSimulation=off  OutputType=Magnitude  PSBequivalent=0
  Vdc 1 : powerlib/Measurements/Voltage Measurement  Tag=PoWeRsYsTeMmEaSuReMeNt  PhasorSimulation=off  OutputType=Magnitude  PSBequivalent=0
  ref : Subsystem
  B + : PMIOPort  Side=Right
  + : PMIOPort  Port=2  Side=Left
  - : PMIOPort  Port=3  Side=Left
  B - : PMIOPort  Port=4  Side=Right
  tag scope: I_ref=global, Idc_bus=global, Vdc_battery=global, Vdc_bus=global, current=global, g_boost=global, g_buck=global
  wires:
  "Vdc "/1 -> Display2/1, [Vdc_bus]
  Vdc 1/1 -> Display3/1, [Vdc_battery]
  Current Measurement2/1 -> Mean/1, [Idc_bus]
  [g_boost] -> Diode6/1
  +ve reference For Buck --> -ve reference For Boost <--/1(buck) -> [g_buck]
  [g_buck] -> Diode5/1
  +ve reference For Buck --> -ve reference For Boost <--/2(boost) -> [g_boost]
  Mean/1 -> Display6/1
  Current Measurement1/1 -> [current], Mean1/1
  Mean1/1 -> Display1/1
  ref/1(ref) -> [I_ref], +ve reference For Buck --> -ve reference For Boost <--/1(I_ref)
  connections:
  +/RConn1 -- Vdc 1/LConn1 -- Current Measurement1/RConn1
  9mH/LConn1 -- Diode5/RConn1 -- Diode6/LConn1
  1200 uF/LConn1 -- "Vdc "/LConn1 -- Current Measurement2/RConn1 -- Diode5/LConn1
  1200uF/LConn1 -- Current Measurement1/LConn1 -- 9mH/RConn1
  Diode6/RConn1 -- "Vdc "/LConn2 -- B -/RConn1 -- 1200 uF/RConn1 -- Vdc 1/LConn2 -- -/RConn1 -- 1200uF/RConn1
  Current Measurement2/LConn1 -- 1mH1/RConn1
  1mH1/LConn1 -- B +/RConn1

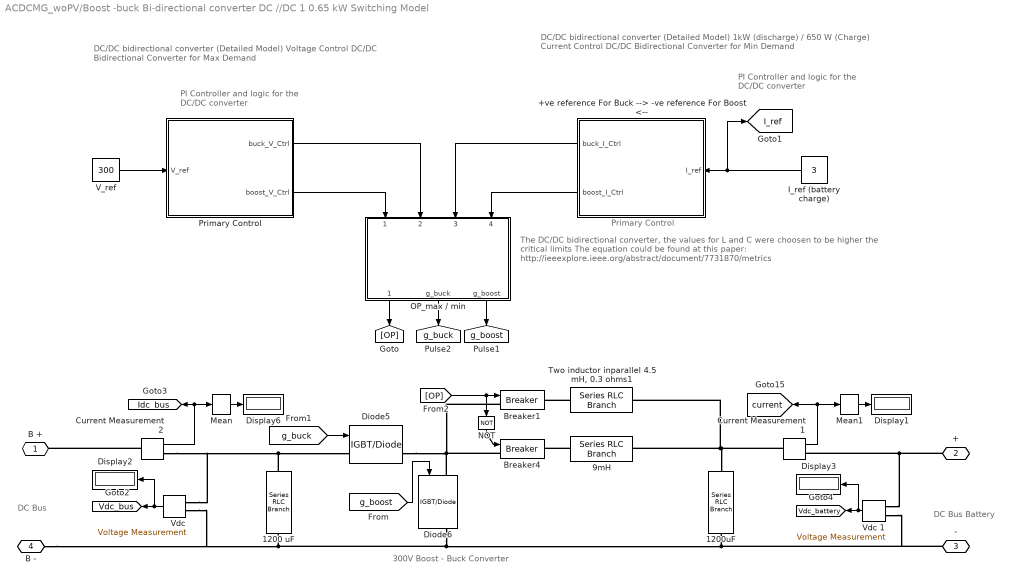
== system ACDCMG_woPV/Boost -buck Bi-directional converter DC //DC 1 0.65 kW Switching Model ==
  note: Primary Control
  note: DC Bus
  note: DC Bus Battery
  note: PI Controller and logic for
      | the DC/DC converter
  note: DC/DC bidirectional converter (Detailed Model)
      | Voltage Control DC/DC Bidirectional Converter for Max Demand
  note: 300V
      | Boost - Buck Converter
  note: PI Controller and logic for
      | the DC/DC converter
  note: DC/DC bidirectional converter (Detailed Model)
      | 1kW (discharge) / 650 W (Charge)
      | Current Control DC/DC Bidirectional Converter for Min Demand
  note: The DC/DC bidirectional converter, the values for L and C were choosen to be higher the critical limits The equation could be found at this paper:
      | http://ieeexplore.ieee.org/abstract/document/7731870/metrics
  +ve reference For Buck --> -ve reference For Boost <-- : Subsystem
      mask Display: image('Icons\FPGA.png');
  1200 uF : powerlib/Elements/Series RLC Branch  LConnTagsString=__new0  RConnTagsString=__new0  BranchType=RC  Resistance=0.1  Inductance=3e-3  SetiL0=off  InitialCurrent=0  Capacitance=1200e-6  Setx0=off  InitialVoltage=150  Measurements=None
  1200uF : powerlib/Elements/Series RLC Branch  LConnTagsString=__new0  RConnTagsString=__new0  BranchType=C  Resistance=1  Inductance=3e-3  SetiL0=off  InitialCurrent=0  Capacitance=1200e-6  Setx0=off  InitialVoltage=130  Measurements=None
  9mH : powerlib/Elements/Series RLC Branch  LConnTagsString=__new0  RConnTagsString=__new0  BranchType=L  Resistance=1  Inductance=9e-3  SetiL0=off  InitialCurrent=0  Capacitance=1e-6  Setx0=off  InitialVoltage=0  Measurements=None
  Breaker1 : powerlib/Elements/Breaker  InitialState=0  SwitchingTimes="[1/60  5/60]"  External=on  BreakerResistance=0.0001  SnubberResistance=1e6  SnubberCapacitance=inf  Measurements=None  MoreParameters=on  NoBreakLoop=off
  Breaker4 : powerlib/Elements/Breaker  InitialState=0  SwitchingTimes="[1/60  5/60]"  External=on  BreakerResistance=0.0001  SnubberResistance=1e6  SnubberCapacitance=inf  Measurements=None  MoreParameters=on  NoBreakLoop=off
  Current Measurement1 : powerlib/Measurements/Current Measurement  PhasorSimulation=off  OutputType=Complex  PSBequivalent=0
  Current Measurement2 : powerlib/Measurements/Current Measurement  PhasorSimulation=off  OutputType=Complex  PSBequivalent=0
  Diode5 : powerlib/Power Electronics/IGBT//Diode  Ron=1e-3  Rs=1e5  Cs=inf  Measurements=on
  Diode6 : powerlib/Power Electronics/IGBT//Diode  Ron=1e-3  Rs=1e5  Cs=inf  Measurements=on
  Display{1..3,6} (4 alike) : Display
  I_ref (battery charge) : Constant  Value=3
  Mean : powerlib_meascontrol/Measurements/Mean  Freq=10  Vinit=0  Ts=0
  Mean1 : powerlib_meascontrol/Measurements/Mean  Freq=10  Vinit=0  Ts=0
  NOT : Logic  Operator=NOT  IconShape=distinctive  AllPortsSameDT=off  OutDataTypeStr=boolean
  OP_max / min : Subsystem
  Primary Control : Subsystem
      mask Display: image('Icons\FPGA.png');
  "Two inductor inparallel 4.5 mH, 0.3 ohms1" : powerlib/Elements/Series RLC Branch  LConnTagsString=__new0  RConnTagsString=__new0  BranchType=RL  Resistance=.25  Inductance=4.5e-3  SetiL0=off  InitialCurrent=0  Capacitance=1e-6  Setx0=off  InitialVoltage=0  Measurements=None
  V_ref : Constant  Value=300
  "Vdc " : powerlib/Measurements/Voltage Measurement  Tag=PoWeRsYsTeMmEaSuReMeNt  PhasorSimulation=off  OutputType=Magnitude  PSBequivalent=0
  Vdc 1 : powerlib/Measurements/Voltage Measurement  Tag=PoWeRsYsTeMmEaSuReMeNt  PhasorSimulation=off  OutputType=Magnitude  PSBequivalent=0
  B + : PMIOPort  Side=Right
  + : PMIOPort  Port=2  Side=Left
  - : PMIOPort  Port=3  Side=Left
  B - : PMIOPort  Port=4  Side=Right
  tag scope: I_ref=global, Idc_bus=global, Vdc_battery=global, Vdc_bus=global, current=global, g_boost=global, g_buck=global
  wires:
  "Vdc "/1 -> Display2/1, [Vdc_bus]
  Vdc 1/1 -> Display3/1, [Vdc_battery]
  Current Measurement2/1 -> Mean/1, [Idc_bus]
  [g_boost] -> Diode6/1
  [g_buck] -> Diode5/1
  Mean/1 -> Display6/1
  Current Measurement1/1 -> [current], Mean1/1
  Mean1/1 -> Display1/1
  V_ref/1 -> Primary Control/1(V_ref)
  OP_max / min/1(Op_Max / Min) -> [OP]
  [OP] -> NOT/1, Breaker1/1
  NOT/1 -> Breaker4/1
  I_ref (battery charge)/1 -> [I_ref], +ve reference For Buck --> -ve reference For Boost <--/1(I_ref)
  +ve reference For Buck --> -ve reference For Boost <--/1(buck_I_Ctrl) -> OP_max / min/3(buck_I_Ctrl)
  +ve reference For Buck --> -ve reference For Boost <--/2(boost_I_Ctrl) -> OP_max / min/4(boost_I_Ctrll)
  OP_max / min/2(g_buck) -> [g_buck]
  OP_max / min/3(g_boost) -> [g_boost]
  Primary Control/1(buck_V_Ctrl) -> OP_max / min/2(buck_V_Ctrl)
  Primary Control/2(boost_V_Ctrl) -> OP_max / min/1(boost_V_Ctrll)
  connections:
  +/RConn1 -- Vdc 1/LConn1 -- Current Measurement1/RConn1
  Diode5/RConn1 -- Breaker1/LConn1 -- Breaker4/LConn1 -- Diode6/LConn1
  1200 uF/LConn1 -- "Vdc "/LConn1 -- Current Measurement2/RConn1 -- Diode5/LConn1
  Diode6/RConn1 -- "Vdc "/LConn2 -- B -/RConn1 -- 1200 uF/RConn1 -- Vdc 1/LConn2 -- -/RConn1 -- 1200uF/RConn1
  Current Measurement2/LConn1 -- B +/RConn1
  "Two inductor inparallel 4.5 mH, 0.3 ohms1"/LConn1 -- Breaker1/RConn1
  Current Measurement1/LConn1 -- 1200uF/LConn1 -- 9mH/RConn1 -- "Two inductor inparallel 4.5 mH, 0.3 ohms1"/RConn1
  9mH/LConn1 -- Breaker4/RConn1
